simulink model "ACT_PROJECT"  (R2023a)
settings: Solver=VariableStepAuto  StartTime=0.0  StopTime=1  RelTol=1e-3
undefined symbols (not defined in the file): Ion, Lithium
libraries: spsBreakerLib x12, spsSeriesRLCBranchLib x9, spsCurrentMeasurementLib x5, spsDiodeLib x5, spsIGBTDiodeLib x4, spsMultimeterLib x4, spsVoltageMeasurementLib x3, spsBatteryLib x2, spsMeanLib x2, spsMosfetLib x1, spsPVArrayLib x1, simulink x1
settings Model: Creator=91638  LastModifiedBy=91638

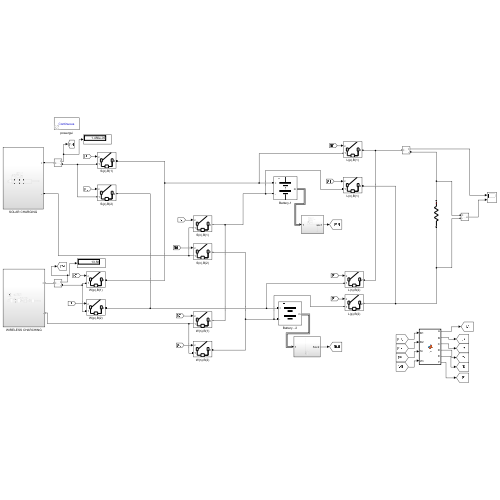
[thumbnail: Simulink's stored preview of the top-level diagram]
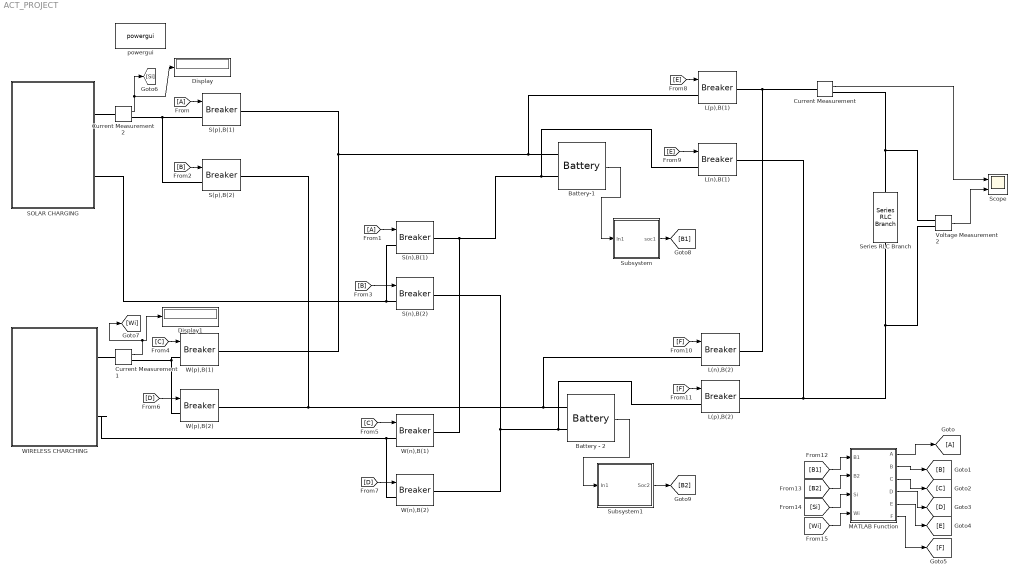
== system ACT_PROJECT ==
  Battery - 2 : spsBatteryLib/Battery  BatType=Lithium-Ion  ShowTempParam=off  ThermalPreset=no  ShowAgeParam=off  NomV=23  NomQ=232  SOC=80  Batt_Tr=0.5  PresetModel=on  MaxQ=232  MinV=17.25  FullV=26.7717  Dis_rate=100.8696  R=0.00099138  Normal_OP=209.8087  expZone="[24.8489      11.3983]"  current=[6.5 13 32.5]  Units=Time  Tci=20  NomT=20  T2=-30  MaxQ2=4.8  FullV2=7.1  Normal_OP2=5.655  expZone2="[6.58           1]"  Rca=0.6  ti=2000  Dp=0  Neq0=0  Tsim=1e6  Ta1=25  Qeol=5.4*0.9  Reol=0.013333*1.2  Char_age=[2.3478, 3]  Dis_age=[2.3478, 10]  N1=1500  N2=10500  N3=1000  N4=1400  Ta2=45  N5=950
  Battery-1 : spsBatteryLib/Battery  BatType=Lithium-Ion  ShowTempParam=off  ThermalPreset=no  ShowAgeParam=off  NomV=23  NomQ=232  SOC=4  Batt_Tr=0.5  PresetModel=on  MaxQ=232  MinV=17.25  FullV=26.7717  Dis_rate=100.8696  R=0.00099138  Normal_OP=209.8087  expZone="[24.8489      11.3983]"  current=[6.5 13 32.5]  Units=Time  Tci=20  NomT=20  T2=-30  MaxQ2=4.8  FullV2=7.1  Normal_OP2=5.655  expZone2="[6.58           1]"  Rca=0.6  ti=2000  Dp=0  Neq0=0  Tsim=1e6  Ta1=25  Qeol=5.4*0.9  Reol=0.013333*1.2  Char_age=[2.3478, 3]  Dis_age=[2.3478, 10]  N1=1500  N2=10500  N3=1000  N4=1400  Ta2=45  N5=950
  Current Measurement : spsCurrentMeasurementLib/Current Measurement  PhasorSimulation=off  OutputType=Complex  PSBequivalent=0
  Current Measurement1 : spsCurrentMeasurementLib/Current Measurement  PhasorSimulation=off  OutputType=Complex  PSBequivalent=0
  Current Measurement2 : spsCurrentMeasurementLib/Current Measurement  PhasorSimulation=off  OutputType=Complex  PSBequivalent=0
  Display : Display
  Display1 : Display
  From : From
  From1 : From
  Goto : Goto
  L(n),B(1) : spsBreakerLib/Breaker  InitialState=0  SwitchingTimes="[1/60  5/60]"  External=on  BreakerResistance=0.01  SnubberResistance=1e6  SnubberCapacitance=inf  Measurements=None  MoreParameters=on  NoBreakLoop=off
  L(n),B(2) : spsBreakerLib/Breaker  InitialState=0  SwitchingTimes="[1/60  5/60]"  External=on  BreakerResistance=0.01  SnubberResistance=1e6  SnubberCapacitance=inf  Measurements=None  MoreParameters=on  NoBreakLoop=off
  L(p),B(1) : spsBreakerLib/Breaker  InitialState=0  SwitchingTimes="[1/60  5/60]"  External=on  BreakerResistance=0.01  SnubberResistance=1e6  SnubberCapacitance=inf  Measurements=None  MoreParameters=on  NoBreakLoop=off
  L(p),B(2) : spsBreakerLib/Breaker  InitialState=0  SwitchingTimes="[1/60  5/60]"  External=on  BreakerResistance=0.01  SnubberResistance=1e6  SnubberCapacitance=inf  Measurements=None  MoreParameters=on  NoBreakLoop=off
  MATLAB Function : MATLAB Function  TreatAsAtomicUnit=on
  S(n),B(1) : spsBreakerLib/Breaker  InitialState=0  SwitchingTimes="[1/60  5/60]"  External=on  BreakerResistance=0.01  SnubberResistance=1e6  SnubberCapacitance=inf  Measurements=None  MoreParameters=on  NoBreakLoop=off
  S(n),B(2) : spsBreakerLib/Breaker  InitialState=0  SwitchingTimes="[1/60  5/60]"  External=on  BreakerResistance=0.01  SnubberResistance=1e6  SnubberCapacitance=inf  Measurements=None  MoreParameters=on  NoBreakLoop=off
  S(p),B(1) : spsBreakerLib/Breaker  InitialState=0  SwitchingTimes="[1/60  5/60]"  External=on  BreakerResistance=0.01  SnubberResistance=1e6  SnubberCapacitance=inf  Measurements=None  MoreParameters=on  NoBreakLoop=off
  S(p),B(2) : spsBreakerLib/Breaker  InitialState=0  SwitchingTimes="[1/60  5/60]"  External=on  BreakerResistance=0.01  SnubberResistance=1e6  SnubberCapacitance=inf  Measurements=None  MoreParameters=on  NoBreakLoop=off
  SOLAR CHARGING : Subsystem
  Scope : Scope  NumInputPorts=2
  Series RLC Branch : spsSeriesRLCBranchLib/Series RLC Branch  LConnTagsString=__new0  RConnTagsString=__new0  BranchType=R  Resistance=100  Inductance=1e-3  SetiL0=off  InitialCurrent=0  Capacitance=1e-6  Setx0=off  InitialVoltage=0  Measurements=None
  Subsystem : Subsystem
  Subsystem1 : Subsystem
  Voltage Measurement2 : spsVoltageMeasurementLib/Voltage Measurement  PhasorSimulation=off  OutputType=Complex  PSBequivalent=0
  W(n),B(1) : spsBreakerLib/Breaker  InitialState=0  SwitchingTimes="[1/60  5/60]"  External=on  BreakerResistance=0.01  SnubberResistance=1e6  SnubberCapacitance=inf  Measurements=None  MoreParameters=on  NoBreakLoop=off
  W(n),B(2) : spsBreakerLib/Breaker  InitialState=0  SwitchingTimes="[1/60  5/60]"  External=on  BreakerResistance=0.01  SnubberResistance=1e6  SnubberCapacitance=inf  Measurements=None  MoreParameters=on  NoBreakLoop=off
  W(p),B(1) : spsBreakerLib/Breaker  InitialState=0  SwitchingTimes="[1/60  5/60]"  External=on  BreakerResistance=0.01  SnubberResistance=1e6  SnubberCapacitance=inf  Measurements=None  MoreParameters=on  NoBreakLoop=off
  W(p),B(2) : spsBreakerLib/Breaker  InitialState=0  SwitchingTimes="[1/60  5/60]"  External=on  BreakerResistance=0.01  SnubberResistance=1e6  SnubberCapacitance=inf  Measurements=None  MoreParameters=on  NoBreakLoop=off
  WIRELESS CHARCHING : Subsystem
  powergui : spspowerguiLib/powergui  Priority=1  SimulationMode=Continuous  SampleTime=50e-6  frequency=60  Iterations=50  frequencyindice=0  Pbase=100e6  ErrMax=1e-4  UnitsV=kV  UnitsW=MW  buscounter=0  FunctionMessages=off  echomessages=off  EnableUseOfTLC=off  CurrentSourceSwitches=off  DisableSnubberDevices=off  DisableRonSwitches=off  DisableVfSwitches=off  DisplayEquations=off  AutomaticDiscreteSolvers=off  SolverType=Tustin/Backward Euler (TBE)  Interpol=off  ExternalGateDelay=off  methode=off  Ts=100  x0status=blocks  SPID=on  SwTol=0  HookPort=off  NonlinearTolerance=1e-4  nMaxIteration=100  ContinueOnMaxIteration=off  RestoreLinks=warning  ResistiveCurrentMeasurement=off  Frange=[0:2:500]  Ylog=off  Xlog=on  ShowGrid=off  save=off  variable=ZData  structure=source  ZoomFFT=off  StartTime=0.1  cycles=5  DisplayStyle=2  fundamental=50  FreqAxis=on  MaxFrequency=1000  frequencyindicesteady=1  RmsSteady=1  display=off
  wires:
  Battery-1/1 -> Subsystem/1(In1)
  Battery - 2/1 -> Subsystem1/1(In1)
  Current Measurement/1 -> Scope/1
  Voltage Measurement2/1 -> Scope/2
  [E] -> L(n),B(1)/1
  [E] -> L(p),B(1)/1
  [F] -> L(n),B(2)/1
  [F] -> L(p),B(2)/1
  [C] -> W(n),B(1)/1
  [D] -> W(n),B(2)/1
  [D] -> W(p),B(2)/1
  [C] -> W(p),B(1)/1
  [B] -> S(p),B(2)/1
  From/1 -> S(p),B(1)/1
  [B] -> S(n),B(2)/1
  From1/1 -> S(n),B(1)/1
  MATLAB Function/5(E) -> [E]
  MATLAB Function/3(C) -> [C]
  MATLAB Function/1(A) -> Goto/1
  [Wi] -> MATLAB Function/4(Wi)
  MATLAB Function/2(B) -> [B]
  MATLAB Function/4(D) -> [D]
  MATLAB Function/6(F) -> [F]
  [B2] -> MATLAB Function/2(B2)
  [Si] -> MATLAB Function/3(Si)
  [B1] -> MATLAB Function/1(B1)
  Current Measurement2/1 -> Display/1, [Si]
  Subsystem/1(soc1) -> [B1]
  Subsystem1/1(Soc2) -> [B2]
  Current Measurement1/1 -> [Wi], Display1/1
  connections:
  Current Measurement2/LConn1 -- SOLAR CHARGING/RConn1
  S(p),B(1)/RConn1 -- W(p),B(1)/RConn1 -- L(p),B(1)/LConn1 -- Battery-1/LConn1
  W(p),B(2)/LConn1 -- W(p),B(1)/LConn1 -- Current Measurement1/RConn1
  S(p),B(2)/RConn1 -- W(p),B(2)/RConn1 -- L(n),B(2)/LConn1 -- Battery - 2/LConn1
  Voltage Measurement2/LConn1 -- Current Measurement/RConn1 -- Series RLC Branch/LConn1
  S(n),B(2)/LConn1 -- SOLAR CHARGING/RConn2 -- S(n),B(1)/LConn1
  Battery-1/LConn2 -- S(n),B(1)/RConn1 -- W(n),B(1)/RConn1 -- L(n),B(1)/LConn1
  WIRELESS CHARCHING/RConn2 -- W(n),B(1)/LConn1 -- W(n),B(2)/LConn1
  L(n),B(1)/RConn1 -- Voltage Measurement2/LConn2 -- Series RLC Branch/RConn1 -- L(p),B(2)/RConn1
  L(p),B(2)/LConn1 -- S(n),B(2)/RConn1 -- W(n),B(2)/RConn1 -- Battery - 2/LConn2
  L(p),B(1)/RConn1 -- L(n),B(2)/RConn1 -- Current Measurement/LConn1
  WIRELESS CHARCHING/RConn1 -- Current Measurement1/LConn1
  Current Measurement2/RConn1 -- S(p),B(2)/LConn1 -- S(p),B(1)/LConn1

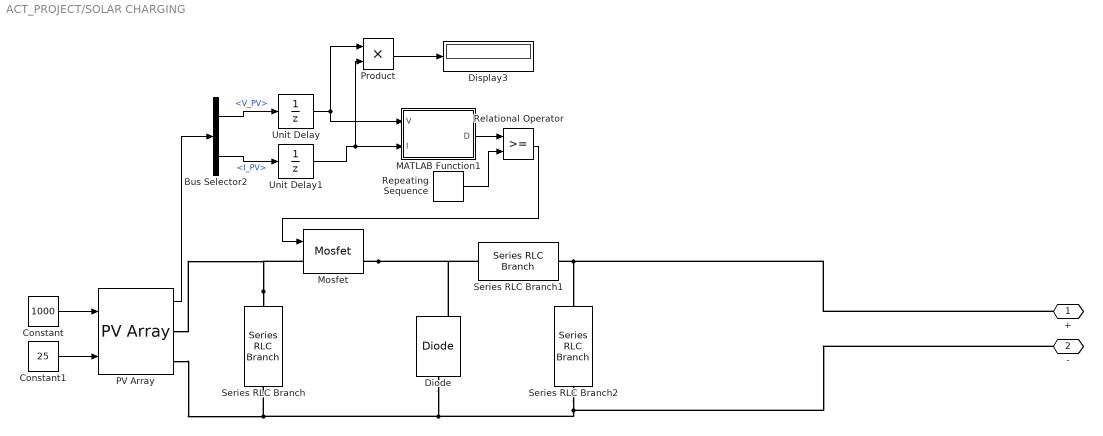
== system ACT_PROJECT/SOLAR CHARGING ==
  Bus Selector2 : BusSelector  OutputSignals=V_PV,I_PV
  Constant : Constant  Value=1000
  Constant1 : Constant  Value=25
  Diode : spsDiodeLib/Diode  Ron=0.001  Lon=0  Vf=0.8  IC=0  UseSnubber=0  Rs=500  Cs=250e-9  Measurements=on
  Display3 : Display
  MATLAB Function1 : MATLAB Function  TreatAsAtomicUnit=on
  Mosfet : spsMosfetLib/Mosfet  Ron=0.1  Lon=0  Rd=0.01  Vfd=0  IC=0  Rs=1e5  Cs=inf  Measurements=on
  PV Array : spsPVArrayLib/PV Array  Npar=1  Nser=1  PlotType=array @ 25 deg.C & specified irradiances  S_vec="[ 1000  500  100 ]"  Temp_C_vec="[ 45 25  ]"  ModuleName=User-defined  PlotWhenSelected=off  Pm=416  Ncell=60  Voc=36.3  Isc=14  Vm=32  Im=13  beta_Voc_pc=-0.36099  alpha_Isc_pc=0.102  beta_Voc=-0.13104  alpha_Isc=0.01428  IL=14.0001  I0=2.1562e-10  nI=1.0006  Rsh=64.0004  Rs=0.12551  RobustModel=off  RobustCellTemperature=313.3991  BAL=on  Tc=1e-6  Tfilter=5e-5
  Product : Product
  Relational Operator : RelationalOperator  OutDataTypeStr=boolean  RndMeth=Simplest  InputSameDT=off
  Repeating Sequence : simulink/Sources/Repeating Sequence  rep_seq_t=[0 0.0002]  rep_seq_y=[0 1]
  Series RLC Branch : spsSeriesRLCBranchLib/Series RLC Branch  LConnTagsString=__new0  RConnTagsString=__new0  BranchType=RC  Resistance=0.0001  Inductance=1e-3  SetiL0=off  InitialCurrent=0  Capacitance=1000e-6  Setx0=off  InitialVoltage=0  Measurements=None
  Series RLC Branch1 : spsSeriesRLCBranchLib/Series RLC Branch  LConnTagsString=__new0  RConnTagsString=__new0  BranchType=L  Resistance=1  Inductance=0.7393e-3  SetiL0=off  InitialCurrent=0  Capacitance=1e-6  Setx0=off  InitialVoltage=0  Measurements=None
  Series RLC Branch2 : spsSeriesRLCBranchLib/Series RLC Branch  LConnTagsString=__new0  RConnTagsString=__new0  BranchType=C  Resistance=1  Inductance=1e-3  SetiL0=off  InitialCurrent=0  Capacitance=190.217e-6  Setx0=off  InitialVoltage=0  Measurements=None
  Unit Delay : UnitDelay  SampleTime=-1  HasFrameUpgradeWarning=on
  Unit Delay1 : UnitDelay  SampleTime=-1  HasFrameUpgradeWarning=on
  + : PMIOPort  Side=Right
  - : PMIOPort  Port=2  Side=Right
  wires:
  Unit Delay1/1 -> MATLAB Function1/2(I), Product/2
  Bus Selector2/1 -> Unit Delay/1  "<V_PV>"
  MATLAB Function1/1(D) -> Relational Operator/1
  Repeating Sequence/1 -> Relational Operator/2
  Unit Delay/1 -> MATLAB Function1/1(V), Product/1
  Bus Selector2/2 -> Unit Delay1/1  "<I_PV>"
  Constant1/1 -> PV Array/2
  PV Array/1 -> Bus Selector2/1
  Relational Operator/1 -> Mosfet/1
  Constant/1 -> PV Array/1
  Product/1 -> Display3/1
  connections:
  Mosfet/RConn1 -- Diode/RConn1 -- Series RLC Branch1/LConn1
  Series RLC Branch2/RConn1 -- -/RConn1 -- PV Array/RConn2 -- Series RLC Branch/RConn1 -- Diode/LConn1
  Series RLC Branch/LConn1 -- PV Array/RConn1 -- Mosfet/LConn1
  Series RLC Branch1/RConn1 -- +/RConn1 -- Series RLC Branch2/LConn1

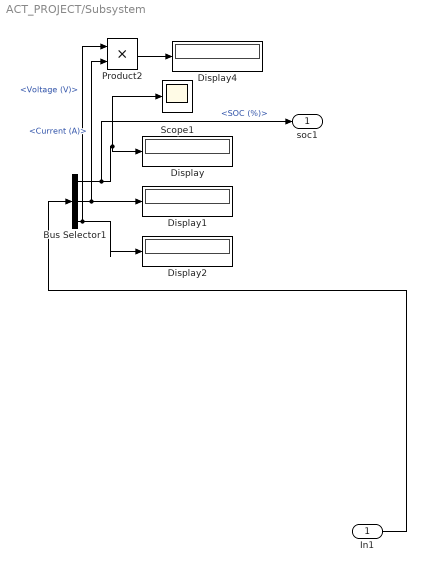
== system ACT_PROJECT/Subsystem ==
  In1 : Inport
  Bus Selector1 : BusSelector  OutputSignals=SOC (%),Current (A),Voltage (V)
  Display{,1..2,4} (4 alike) : Display
  Product2 : Product
  Scope1 : Scope
  soc1 : Outport
  wires:
  Bus Selector1/2 -> Display1/1, Product2/2  "<Current (A)>"
  Bus Selector1/3 -> Display2/1, Product2/1  "<Voltage (V)>"
  In1/1 -> Bus Selector1/1
  Product2/1 -> Display4/1
  Bus Selector1/1 -> soc1/1, Scope1/1, Display/1  "<SOC (%)>"

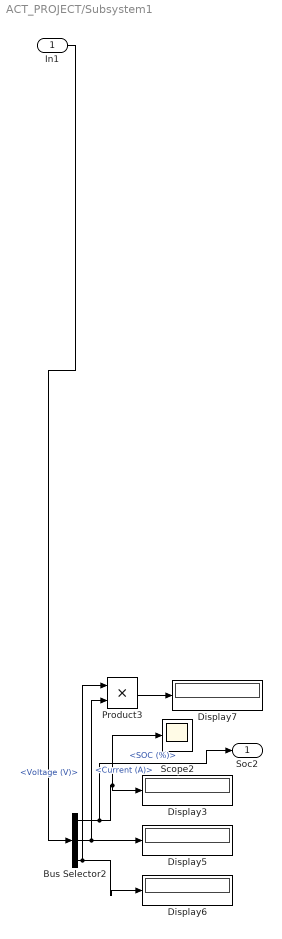
== system ACT_PROJECT/Subsystem1 ==
  In1 : Inport
  Bus Selector2 : BusSelector  OutputSignals=SOC (%),Current (A),Voltage (V)
  Display{3,5..7} (4 alike) : Display
  Product3 : Product
  Scope2 : Scope
  Soc2 : Outport
  wires:
  Bus Selector2/2 -> Display5/1, Product3/2  "<Current (A)>"
  Bus Selector2/3 -> Display6/1, Product3/1  "<Voltage (V)>"
  Bus Selector2/1 -> Soc2/1, Scope2/1, Display3/1  "<SOC (%)>"
  Product3/1 -> Display7/1
  In1/1 -> Bus Selector2/1

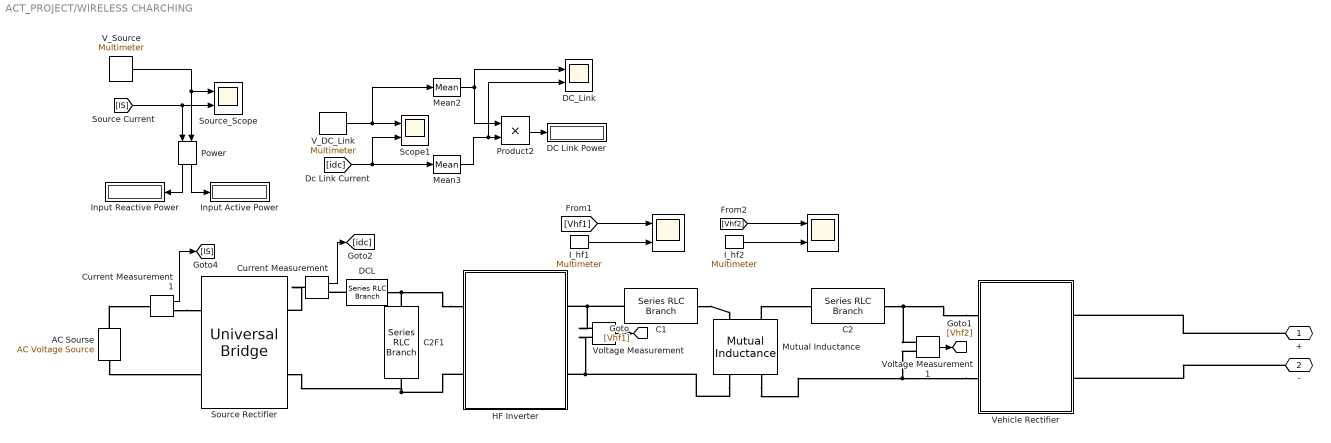
== system ACT_PROJECT/WIRELESS CHARCHING ==
  " " : Scope  NumInputPorts=2
  "   " : Scope  NumInputPorts=2
  AC Sourse : spsACVoltageSourceLib/AC Voltage Source  Amplitude=325  Phase=0  Frequency=50  SampleTime=0  Measurements=Voltage  BusType=swing  Pref=10e3  Qref=0  Qmin=-inf  Qmax=+inf
  C1 : spsSeriesRLCBranchLib/Series RLC Branch  LConnTagsString=__new0  RConnTagsString=__new0  BranchType=C  Resistance=1e-6  Inductance=1e-3  SetiL0=off  InitialCurrent=0  Capacitance=105.74e-9  Setx0=off  InitialVoltage=0  Measurements=Branch current
  C2 : spsSeriesRLCBranchLib/Series RLC Branch  LConnTagsString=__new0  RConnTagsString=__new0  BranchType=C  Resistance=1e-6  Inductance=1e-3  SetiL0=off  InitialCurrent=0  Capacitance=109.69e-9  Setx0=off  InitialVoltage=0  Measurements=Branch current
  C2F1 : spsSeriesRLCBranchLib/Series RLC Branch  LConnTagsString=__new0  RConnTagsString=__new0  BranchType=C  Resistance=1e-6  Inductance=1e-3  SetiL0=off  InitialCurrent=0  Capacitance=300e-6  Setx0=off  InitialVoltage=0  Measurements=None
  Current Measurement : spsCurrentMeasurementLib/Current Measurement  PhasorSimulation=off  OutputType=Complex  PSBequivalent=0
  Current Measurement1 : spsCurrentMeasurementLib/Current Measurement  PhasorSimulation=off  OutputType=Complex  PSBequivalent=0
  DC Link Power : Display
  DCL : spsSeriesRLCBranchLib/Series RLC Branch  LConnTagsString=__new0  RConnTagsString=__new0  BranchType=L  Resistance=0.1  Inductance=10e-3  SetiL0=off  InitialCurrent=0  Capacitance=1e-6  Setx0=off  InitialVoltage=0  Measurements=Branch current
  DC_Link : Scope  NumInputPorts=2
  HF Inverter : Subsystem
  I_hf1 : spsMultimeterLib/Multimeter  L=15  sel=9  yselected={}  Gain=1  OutputType=Complex  PlotAtSimulationStop=off  PhasorSimulation=off
  I_hf2 : spsMultimeterLib/Multimeter  L=15  sel=10  yselected={}  Gain=1  OutputType=Complex  PlotAtSimulationStop=off  PhasorSimulation=off
  Input Active Power : Display
  Input Reactive Power : Display
  Mean2 : spsMeanLib/Mean  Freq=50  Vinit=0  Ts=0
  Mean3 : spsMeanLib/Mean  Freq=50  Vinit=0  Ts=0
  Mutual Inductance : spsMutualInductanceLib/Mutual Inductance  LConnTagsString=a|b  RConnTagsString=A|B  TypeOfMutual=Two or three windings with equal mutual terms  NumberOfWindings=3  SelfImpedance1=[1e-3 266.16e-6]  SelfImpedance2=[1e-3 256.79e-6]  ThreeWindings=off  SelfImpedance3=[ 1.1 1.1e-03]  MutualImpedance=[0 85.46e-6]  InductanceMatrix="[1.0 0.9  0.9 ;  0.9 1.0  0.9;  0.9 0.9 1.0 ] * 1e-3"  ResistanceMatrix="[1.0 0.9  0.9 ;  0.9 1.0  0.9;  0.9 0.9 1.0 ]"  Measurements=None
  Power : spsPowerLib/Power  Freq=50  Vinit=[1, 0]  Iinit=[1, 0]  Ts=0
  Product2 : Product
  Scope1 : Scope  NumInputPorts=2
  Source Rectifier : spsUniversalBridgeLib/Universal Bridge  Arms=2  SnubberResistance=1e5  SnubberCapacitance=inf  Device=Diodes  Ron=1e-3  Lon=0  ForwardVoltages="[  0  0  ]"  ForwardVoltage=0  GTOparameters=[ 10e-6 , 20e-6 ]  IGBTparameters=[ 1e-6 , 2e-6 ]  Measurements=All voltages and currents  Measurements_2=None  converterType=Rectifier
  Source_Scope : Scope  NumInputPorts=2
  V_DC_Link : spsMultimeterLib/Multimeter  L=15  sel=7  yselected={}  Gain=1  OutputType=Complex  PlotAtSimulationStop=off  PhasorSimulation=off
  V_Source : spsMultimeterLib/Multimeter  L=15  sel=8  yselected={}  Gain=1  OutputType=Complex  PlotAtSimulationStop=off  PhasorSimulation=off
  Vehicle Rectifier : Subsystem
  Voltage Measurement : spsVoltageMeasurementLib/Voltage Measurement  PhasorSimulation=off  OutputType=Complex  PSBequivalent=0
  Voltage Measurement1 : spsVoltageMeasurementLib/Voltage Measurement  PhasorSimulation=off  OutputType=Complex  PSBequivalent=0
  + : PMIOPort  Side=Right
  - : PMIOPort  Port=2  Side=Right
  wires:
  V_Source/1 -> Source_Scope/1, Power/1
  V_DC_Link/1 -> Mean2/1, Scope1/1
  Mean3/1 -> DC_Link/2, Product2/2
  [Vhf1] -> " "/1
  [idc] -> Mean3/1, Scope1/2
  [Vhf2] -> "   "/1
  Voltage Measurement1/1 -> [Vhf2]
  Power/1 -> Input Active Power/1
  Mean2/1 -> DC_Link/1, Product2/1
  Product2/1 -> DC Link Power/1
  [IS] -> Power/2, Source_Scope/2
  I_hf1/1 -> " "/2
  Current Measurement/1 -> [idc]
  Voltage Measurement/1 -> [Vhf1]
  Power/2 -> Input Reactive Power/1
  I_hf2/1 -> "   "/2
  Current Measurement1/1 -> [IS]
  connections:
  C2F1/RConn1 -- Source Rectifier/RConn2 -- HF Inverter/LConn2
  -/RConn1 -- Vehicle Rectifier/RConn2
  HF Inverter/RConn1 -- C1/LConn1 -- Voltage Measurement/LConn1
  HF Inverter/LConn1 -- C2F1/LConn1 -- DCL/LConn1
  AC Sourse/RConn1 -- Current Measurement1/LConn1
  HF Inverter/RConn2 -- Mutual Inductance/RConn1 -- Voltage Measurement/LConn2
  Vehicle Rectifier/LConn1 -- C2/RConn1 -- Voltage Measurement1/LConn1
  DCL/RConn1 -- Current Measurement/RConn1
  Current Measurement/LConn1 -- Source Rectifier/RConn1
  C1/RConn1 -- Mutual Inductance/LConn1
  AC Sourse/LConn1 -- Source Rectifier/LConn2
  Vehicle Rectifier/LConn2 -- Mutual Inductance/RConn2 -- Voltage Measurement1/LConn2
  Mutual Inductance/LConn2 -- C2/LConn1
  +/RConn1 -- Vehicle Rectifier/RConn1
  Current Measurement1/RConn1 -- Source Rectifier/LConn1

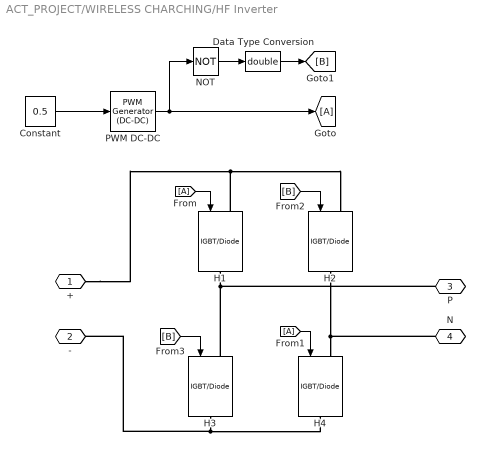
== system ACT_PROJECT/WIRELESS CHARCHING/HF Inverter ==
  Constant : Constant  Value=0.5
  Data Type Conversion : DataTypeConversion  OutDataTypeStr=double  SaturateOnIntegerOverflow=off  RndMeth=Floor
  From : From
  From1 : From
  Goto : Goto
  H{1..4} (4 alike) : spsIGBTDiodeLib/IGBT//Diode  Ron=1e-3  Rs=1e5  Cs=inf  Measurements=off
  "NOT " : Logic  Operator=NOT  IconShape=distinctive  AllPortsSameDT=off  OutDataTypeStr=boolean
  PWM DC-DC : spsPWMGeneratorDCDCLib/PWM Generator (DC-DC)  Fsw=30000  Ts=0
  + : PMIOPort  Side=Left
  - : PMIOPort  Port=2  Side=Left
  P : PMIOPort  Port=3  Side=Right
  N : PMIOPort  Port=4  Side=Right
  wires:
  [B] -> H2/1
  [B] -> H3/1
  From1/1 -> H4/1
  From/1 -> H1/1
  "NOT "/1 -> Data Type Conversion/1
  Constant/1 -> PWM DC-DC/1
  Data Type Conversion/1 -> [B]
  PWM DC-DC/1 -> "NOT "/1, Goto/1
  connections:
  H1/LConn1 -- H2/LConn1 -- +/RConn1
  H2/RConn1 -- N/RConn1 -- H4/LConn1
  H3/RConn1 -- -/RConn1 -- H4/RConn1
  H3/LConn1 -- P/RConn1 -- H1/RConn1

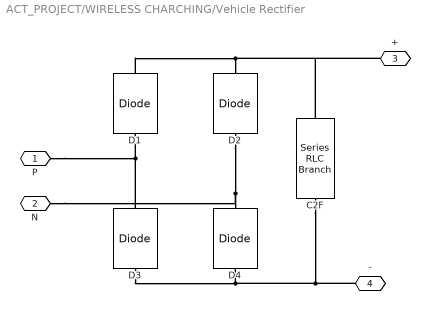
== system ACT_PROJECT/WIRELESS CHARCHING/Vehicle Rectifier ==
  C2F : spsSeriesRLCBranchLib/Series RLC Branch  LConnTagsString=__new0  RConnTagsString=__new0  BranchType=C  Resistance=1e-6  Inductance=1e-3  SetiL0=off  InitialCurrent=0  Capacitance=300e-6  Setx0=off  InitialVoltage=0  Measurements=Branch voltage
  D{1..4} (4 alike) : spsDiodeLib/Diode  Ron=0.001  Lon=0  Vf=0.8  IC=0  UseSnubber=0  Rs=500  Cs=250e-9  Measurements=off
  P : PMIOPort  Side=Left
  N : PMIOPort  Port=2  Side=Left
  + : PMIOPort  Port=3  Side=Right
  - : PMIOPort  Port=4  Side=Right
  connections:
  D1/RConn1 -- +/RConn1 -- C2F/LConn1 -- D2/RConn1
  D3/RConn1 -- P/RConn1 -- D1/LConn1
  C2F/RConn1 -- -/RConn1 -- D3/LConn1 -- D4/LConn1
  D2/LConn1 -- N/RConn1 -- D4/RConn1

== matlab function ACT_PROJECT/SOLAR CHARGING/MATLAB Function1 ==
  data: V input; D output; I input
function D = DutyRatio(V, I)

Dmax = 0.95;
Dmin = 0;
Dinit = 0.95;
deltaD = 0.0001;
persistent Vold Pold Dold;
persistent atMPP;  % A flag to track whether at the MPP

dataType = 'double';

if isempty(Vold)
    Vold = 0;
    Pold = 0;
    Dold = Dinit;
    atMPP = false;
end

P = V * I;
dV = V - Vold;
dP = P - Pold;

if ~atMPP  % Continue adjusting only if not at the MPP
    if dP ~= 0
        if dP < 0
            if dV < 0
                D = Dold - deltaD;
            else
                D = Dold + deltaD;
            end
        else
            if dV < 0
                D = Dold + deltaD;
            else
                D = Dold - deltaD;
            end
        end
    else
        D = Dold;
    end

    if D >= Dmax || D <= Dmin
        D = Dold;
    end
    
    % Check for convergence (near MPP)
    if abs(P - Pold) < 0.01
        atMPP = true;
    end
else
    % If at MPP, keep the duty ratio unchanged
    D = Dold;
end

% Update persistent variables
Dold = D;
Vold = V;
Pold = P;

== matlab function ACT_PROJECT/MATLAB Function ==
  data: B1 input; A output; B2 input; Si input; Wi input; B output; C output; D output; E output; F output
function [A,B,C,D,E,F]= fcn(B1,B2,Si,Wi)

%initializing the breaker conditions
A=0;
B=0;
C=0;
D=0;
E=0;
F=0;

if B1>=5 || B2<=1
    E=1;
    F=0;
    if Si>=Wi
        A=0;
        B=1;
        C=0;
        D=0;
    else
        A=0;
        B=0;
        C=0;
        D=1;
    end
else
    E=0;
    F=1;
    if Si>=Wi
        A=1;
        B=0;
        C=0;
        D=0;
    else
        A=0;
        B=0;
        C=1;
        D=0;
    end
end
